simulink model "mrc"  (R2014a)
settings: Solver=ode45  StartTime=0.0  StopTime=10.0  RelTol=1e-3
InitFcn:
  | % Bunlar 3 boyutlu sistemler içindir.
  | % Farklı boyut için bazı düzenlemeler gerekir.
  | A=[-3 -1 -1;
  |        8  3  3;
  |     -20 -10 -1];
  | B=[2;-1;5];
  | Qc=[B, A*B, A*A*B];
  | lmd1=-5; lmd2=-6+4i; lmd3=-6-4i;
  | alfap=poly([lmd1 lmd2 lmd3]);
  | alfa=alfap(end:-1:2);  % alfa(1) aslında alfa0
  | ap=poly(A);
  | a=ap(end:-1:2);  % a(1) aslında a0
  | Kcr=alfa-a;
  | Bcr=[0;0;1];
  | T(1,:)=Bcr'*inv(Qc);
  | T(2,:)=T(1,:)*A;
  | T(3,:)=T(2,:)*A;
  | K=Kcr*T;
settings Model: Creator=Ata  LastModifiedBy=Ata

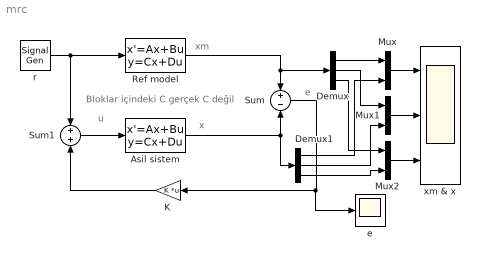
== system mrc ==
  note: u
  note: x
  note: e
  note: Bloklar içindeki C gerçek C değil
  note: xm
  Asil sistem : StateSpace  A=A  B=B  C=eye(3)  D=zeros(3,1)  X0=[0;0;0]
  Demux : Demux  Outputs=3
  Demux1 : Demux  Outputs=3
  K : Gain  Gain=K  Multiplication=Matrix(K*u)
  Mux : Mux  Inputs=2
  Mux1 : Mux  Inputs=2
  Mux2 : Mux  Inputs=2
  Ref model : StateSpace  A=A  B=B  C=eye(3)  D=zeros(3,1)  X0=[20;30;50]
  Sum : Sum  Inputs=+|-
  Sum1 : Sum  Inputs=+|+
  e : Scope
  r : SignalGenerator  Units=rad/sec
  xm & x : Scope  NumInputPorts=3
      settings: YMin=-5~-5~-5  YMax=5~5~5
  wires:
  r/1 -> Sum1/1, Ref model/1
  Ref model/1 -> Demux/1, Sum/1
  Asil sistem/1 -> Demux1/1, Sum/2
  Sum/1 -> e/1, K/1
  K/1 -> Sum1/2
  Sum1/1 -> Asil sistem/1
  Mux/1 -> xm & x/1
  Mux1/1 -> xm & x/2
  Mux2/1 -> xm & x/3
  Demux/1 -> Mux/1
  Demux/2 -> Mux1/1
  Demux/3 -> Mux2/1
  Demux1/1 -> Mux/2
  Demux1/2 -> Mux1/2
  Demux1/3 -> Mux2/2
